simulink library "thermochemical"  (R2017b)
settings: Solver=VariableStepAuto  StartTime=0.0  StopTime=10.0  RelTol=1e-3
values from neighbouring files (symbols this model uses):
  c = conversion_factors()    [blk_clausius_clapeyron.m]    (also in blk_clausius_clapeyron_no_popup.m; blk_cold_room_closed_dry_air.m; blk_reactor_BaCl2_NH3_no_walls.m; blk_reactor_BaCl2_NH3_no_walls_state_space.m)
  cp = metal.cp    [blk_wall_simple.m]    (also in get_metal_properties.m = 390)
  fluid = get_param(blk,'fluid')    [blk_thermodynamic_properties_nonsaturated.m]    (also in blk_thermodynamic_properties_nonsaturated_interpreted.m; blk_thermodynamic_properties_saturated.m; blk_thermodynamic_properties_saturated_interpreted.m; blk_thermodynamic_properties_saturated_mix.m)
  gas = get_material_properties(x.gasName)    [blk_reactor_BaCl2_NH3_cylindrical_no_walls_fun1.m]
  h = get_param(gcb,'ObjectParameters')    [get_param_eval.m]
  rho = metal.rho    [blk_wall_simple.m]    (also in get_metal_properties.m = 8940)
  s = solve(eq,dx,'ReturnConditions',true)    [LMTD_inv.m]    (also in blk_wall_simple.m = get_param_eval(blk,'s'))
  u_gas_at_T_ref = -R * T_ref    [blk_reactor_BaCl2_NH3_no_walls.m]    (also in blk_reactor_BaCl2_NH3_no_walls_state_space.m)
undefined symbols (not defined in the file or in its folder): b_motor, BaCl2, beta, CoolProp, cP_binder, cP_gas, cP_s0, cv, dh_r_0, ENG, heat_exchanger_epsilonNTU_inv_simulink, heat_exchanger_epsilonNTU_simulink, J_motor, K_cin, kappa, Km_motor, La_motor, lookup2D_BreakPoint2, M_binder, N_binder, N_gas_free_volume_init, N_salt, NH3, nh3_v3, nu, P, phase, PID_D_motor, PID_I_motor, PID_P_motor, Ra_motor, Reactor_phase, T, T1, T2, T_init, Tr_init, Tr_ref, U_binder_at_Tr_ref, U_salt_at_X0_Tr_ref, Ur_init, V_void, Valve_regime, Vmax_motor, w_init_motor, X_init
libraries: thermochemical x247, simulink x54, dspsigops x3
(part 6 of 12)

== system thermochemical/Walls/Radial thermal resistance (no energy accumulation) ==
  In3 : Inport
  In1 : Inport  Port=2
  In2 : Inport  Port=3
  In4 : Inport  Port=4
  Divide : Product  Inputs=*/
  Divide1 : Product  Inputs=*/
  Gain2 : Gain  Gain=2*pi
  Math Function : Math  Operator=log  SaturateOnIntegerOverflow=on
  Product : Product  Inputs=**
  Out3 : Outport
  wires:
  Math Function/1 -> Divide/1
  Divide1/1 -> Math Function/1
  In1/1 -> Divide1/2  "Dinner (m)"
  In3/1 -> Product/1  "lambda (W/K/m)"
  Divide/1 -> Out3/1  "R (K/W)"
  In2/1 -> Divide1/1  "Douter (m)"
  In4/1 -> Product/2  "L (m)"
  Product/1 -> Gain2/1
  Gain2/1 -> Divide/2

== system thermochemical/Walls/Wall, simple, h as inputs ==
  note: Convective heat transfer.
      | Wall - Inner interface
  note: Wall, internal energy's
      | differential equation
  note: Convective heat transfer.
      | Wall - Outer interface
  In1 : Inport
  In3 : Inport  Port=2
  In2 : Inport  Port=3
  In4 : Inport  Port=4
  Gain1 : Gain  Gain=s
  Gain12 : Gain  Gain=s
  Gain14 : Gain  Gain=1/(e_mm*1e-3*s*rho*cp)
  Initial condition : Constant  Value=Twall_init
  Integrator4 : Integrator  InitialConditionSource=external  InitialCondition=T_init
  Product : Product
  Product1 : Product
  Sum13 : Sum  Inputs=|-+
  Sum15 : Sum  Inputs=-+
  Sum18 : Sum  Inputs=-+|
  Out2 : Outport
  Out1 : Outport  Port=2
  Out3 : Outport  Port=3
  wires:
  Product/1 -> Gain12/1
  In3/1 -> Product/1  "h outer (W/m²/K)"
  Initial condition/1 -> Integrator4/2
  Sum15/1 -> Gain14/1
  In1/1 -> Sum13/1  "T outer (K)"
  Gain12/1 -> Out3/1, Sum15/1  "Q wall → outer (W)"
  Integrator4/1 -> Sum18/1, Sum13/2, Out2/1  "T wall (K)"
  Sum18/1 -> Product1/1
  Gain1/1 -> Sum15/2, Out1/1  "Q inner → wall (W)"
  Sum13/1 -> Product/2
  Gain14/1 -> Integrator4/1  "dT/dt"
  In2/1 -> Sum18/2  "T inner (K)"
  Product1/1 -> Gain1/1
  In4/1 -> Product1/2  "h inner (W/m²/K)"

== system thermochemical/Walls/Wall, tube with//without fins ==
  note: Convective heat transfer.
      | Wall - Outer interface
  note: Internal energy's
      | differential equation
  note: Convective heat transfer.
      | Wall - Inner interface
  In1 : Inport
  In4 : Inport  Port=2
  In2 : Inport  Port=3
  In5 : Inport  Port=4
  Divide : Product  Inputs=*/
  Initial condition : Constant  Value=Tinit
  Integrator4 : Integrator  InitialConditionSource=external  InitialCondition=T_init
  Product : Product  Inputs=3
  Product1 : Product  Inputs=3
  Subsystem : Subsystem
  Subsystem1 : Subsystem
  Subsystem3 : Subsystem
  Sum13 : Sum  Inputs=|-+
  Sum15 : Sum  Inputs=-+
  Sum18 : Sum  Inputs=-+|
  s12 : Constant  Value=L_m
  s13 : Constant  Value=OD_mm
  s14 : Constant  Value=e_mm
  Out2 : Outport
  Out1 : Outport  Port=2
  Out3 : Outport  Port=3
  Out4 : Outport  Port=4
  wires:
  In2/1 -> Sum18/2  "T inner (K)"
  Divide/1 -> Integrator4/1  "dT/dt"
  Sum13/1 -> Product/3
  Product1/1 -> Sum15/2, Out1/1  "Q inner → wall (W)"
  Sum18/1 -> Product1/1
  Integrator4/1 -> Out2/1, Sum13/2, Sum18/1  "T wall (K)"
  Product/1 -> Sum15/1, Out3/1  "Q wall → outer (W)"
  In1/1 -> Sum13/1  "T outer (K)"
  Sum15/1 -> Divide/1  "Q net"
  Initial condition/1 -> Integrator4/2
  Subsystem3/2(Total tube effective finned area (m2)) -> Product/1
  In5/1 -> Product1/2  "h inner (W/m²/K)"
  In4/1 -> Subsystem3/1(In4), Product/2  "h outer (W/m²/K)"
  s13/1 -> Subsystem/1(In1)
  s14/1 -> Subsystem/2(In2)
  s12/1 -> Subsystem/3(In3)
  Subsystem/1(Inner area (m2)) -> Product1/3
  Subsystem1/1((m*Cp) fins + (m*Cp) tube) -> Divide/2
  Subsystem3/1(Total tube effective finned area (m2)1) -> Out4/1  "eta_fin (0..1)"

== system thermochemical/Walls/Wall, tube with//without fins, with internal heat production ==
  note: Convective heat transfer.
      | Wall - Inner interface
  note: Internal energy's
      | differential equation
  note: Convective heat transfer.
      | Wall - Outer interface
  In1 : Inport
  In4 : Inport  Port=2
  In2 : Inport  Port=3
  In5 : Inport  Port=4
  In3 : Inport  Port=5
  Divide : Product  Inputs=*/
  Initial condition : Constant  Value=Tinit
  Integrator4 : Integrator  InitialConditionSource=external  InitialCondition=T_init
  Product : Product  Inputs=3
  Product1 : Product  Inputs=3
  Subsystem : Subsystem
  Subsystem1 : Subsystem
  Subsystem3 : Subsystem
  Sum13 : Sum  Inputs=|-+
  Sum15 : Sum  Inputs=-++
  Sum18 : Sum  Inputs=-+|
  s12 : Constant  Value=L_m
  s13 : Constant  Value=OD_mm
  s14 : Constant  Value=e_mm
  Out2 : Outport
  Out1 : Outport  Port=2
  Out3 : Outport  Port=3
  Out4 : Outport  Port=4
  wires:
  Subsystem3/1(Total tube effective finned area (m2)1) -> Out4/1  "eta_fin (0..1)"
  Subsystem1/1((m*Cp) fins + (m*Cp) tube) -> Divide/2
  Subsystem/1(Inner area (m2)) -> Product1/3
  s12/1 -> Subsystem/3(In3)
  s14/1 -> Subsystem/2(In2)
  s13/1 -> Subsystem/1(In1)
  In4/1 -> Product/2, Subsystem3/1(In4)  "h outer (W/m²/K)"
  In5/1 -> Product1/2  "h inner (W/m²/K)"
  Subsystem3/2(Total tube effective finned area (m2)) -> Product/1
  Initial condition/1 -> Integrator4/2
  Sum15/1 -> Divide/1  "Q net"
  In1/1 -> Sum13/1  "T outer (K)"
  Product/1 -> Sum15/1, Out3/1  "Q wall → outer (W)"
  Integrator4/1 -> Sum18/1, Sum13/2, Out2/1  "T wall (K)"
  Sum18/1 -> Product1/1
  Product1/1 -> Sum15/3, Out1/1  "Q inner → wall (W)"
  Sum13/1 -> Product/3
  Divide/1 -> Integrator4/1  "dT/dt"
  In2/1 -> Sum18/2  "T inner (K)"
  In3/1 -> Sum15/2  "Q production (W)"

== system thermochemical/Compression/Gas compressor without motor/Compressor's power dW ==
  In1 : Inport
  In7 : Inport  Port=2
  In2 : Inport  Port=3
  Divide1 : Product  Inputs=**
  Sum2 : Sum  Inputs=-+
  Out2 : Outport
  wires:
  Sum2/1 -> Divide1/1  "delta h"
  In1/1 -> Sum2/2  "h_out (J/mol)"
  In7/1 -> Sum2/1  "h_in (J/mol)"
  In2/1 -> Divide1/2  "dn (mol/sec)"
  Divide1/1 -> Out2/1  "dW/dt compr. (W)"

== system thermochemical/Compression/Gas compressor without motor/Cp//Cv ==
  In1 : Inport
  In2 : Inport  Port=2
  Divide : Product  Inputs=*/
  Thermodynamic property (non-saturated) : thermochemical/Thermodynamic fluid properties/Thermodynamic  property (non-saturated)  sel=cp(T,P)  fluid=fluid  reciprocVar=-1  lookup2D_BreakPoint1=fluid.no_sat.T_P_indep.var_indep.T  lookup2D_BreakPoint2=fluid.no_sat.T_P_indep.var_indep.P  lookup2D_Data=fluid.no_sat.T_P_indep.var_dep.Cp_molar
      settings: SourceProductName=@ Thermochemical
  Thermodynamic property (non-saturated)1 : thermochemical/Thermodynamic fluid properties/Thermodynamic  property (non-saturated)  sel=cv(T,P)  fluid=fluid  reciprocVar=-1  lookup2D_BreakPoint1=fluid.no_sat.T_P_indep.var_indep.T  lookup2D_BreakPoint2=fluid.no_sat.T_P_indep.var_indep.P  lookup2D_Data=fluid.no_sat.T_P_indep.var_dep.Cv_molar
      settings: SourceProductName=@ Thermochemical
  Out1 : Outport
  wires:
  Thermodynamic property (non-saturated)/1 -> Divide/1
  Divide/1 -> Out1/1  "gamma (1)"
  In1/1 -> Thermodynamic property (non-saturated)1/1, Thermodynamic property (non-saturated)/1  "T (K)"
  Thermodynamic property (non-saturated)1/1 -> Divide/2
  In2/1 -> Thermodynamic property (non-saturated)1/2, Thermodynamic property (non-saturated)/2  "P (bar)"

== system thermochemical/Compression/Gas compressor without motor/Gas flow rate ==
  In2 : Inport
  In7 : Inport  Port=2
  In1 : Inport  Port=3
  In6 : Inport  Port=4
  Divide2 : Product  Inputs=**
  Divide3 : Product  Inputs=**
  Gain : Gain  Gain=3600
  Swept volume per radian (m3/rad) : Gain  Gain=dVswept_m3_h / dVswept_rmp / (2*pi*60)
  Terminator : Terminator
  Thermodynamic property (non-saturated) : thermochemical/Thermodynamic fluid properties/Thermodynamic  property (non-saturated)  sel=rho(T,P)  fluid=fluid  reciprocVar=-1  lookup2D_BreakPoint1=fluid.no_sat.T_P_indep.var_indep.T  lookup2D_BreakPoint2=fluid.no_sat.T_P_indep.var_indep.P  lookup2D_Data=fluid.no_sat.T_P_indep.var_dep.rho_molar
      settings: SourceProductName=@ Thermochemical
  Thermodynamic property (non-saturated)1 : thermochemical/Thermodynamic fluid properties/Thermodynamic  property (non-saturated)  sel=phase(T,P)  fluid=fluid  reciprocVar=-1  lookup2D_BreakPoint1=fluid.no_sat.T_P_indep.var_indep.T  lookup2D_BreakPoint2=fluid.no_sat.T_P_indep.var_indep.P  lookup2D_Data=fluid.no_sat.T_P_indep.var_dep.phase
      settings: SourceProductName=@ Thermochemical
  Out2 : Outport
  Out1 : Outport  Port=2
  Out3 : Outport  Port=3
  Out4 : Outport  Port=4
  wires:
  Divide2/1 -> Out2/1  "dn/dt (mol/sec)"
  In6/1 -> Divide3/2  "eta vol ([0..1])"
  Divide3/1 -> Divide2/1, Out1/1  "dV/dt effective (m3/sec)"
  In1/1 -> Swept volume per radian (m3/rad)/1  "omega (rad/sec)"
  Swept volume per radian (m3/rad)/1 -> Gain/1, Divide3/1, Out3/1  "dV/dt swept (m3/sec)"
  In7/1 -> Thermodynamic property (non-saturated)1/2, Thermodynamic property (non-saturated)/2  "P in (bar)"
  Thermodynamic property (non-saturated)/1 -> Divide2/2  "rho_gas (mol/m3)"
  In2/1 -> Thermodynamic property (non-saturated)1/1, Thermodynamic property (non-saturated)/1  "T in (K)"
  Gain/1 -> Out4/1  "dV/dt swept (m3/h)"
  Thermodynamic property (non-saturated)1/1 -> Terminator/1  "phase"

== system thermochemical/Compression/Gas compressor without motor/Torque  ==
  In5 : Inport
  In8 : Inport  Port=2
  In6 : Inport  Port=3
  In2 : Inport  Port=4
  In7 : Inport  Port=5
  Divide2 : Product  Inputs=****
  Gain5 : Gain  Gain=1/eta_mech
  Sum2 : Sum  Inputs=-+
  Swept volume per radian (m3/rad) : Constant  Value=dVswept_m3_h / dVswept_rmp / (2*pi*60)
  Thermodynamic property (non-saturated) : thermochemical/Thermodynamic fluid properties/Thermodynamic  property (non-saturated)  sel=rho(T,P)  fluid=fluid  reciprocVar=-1  lookup2D_BreakPoint1=fluid.no_sat.T_P_indep.var_indep.T  lookup2D_BreakPoint2=fluid.no_sat.T_P_indep.var_indep.P  lookup2D_Data=fluid.no_sat.T_P_indep.var_dep.rho_molar
      settings: SourceProductName=@ Thermochemical
  Out4 : Outport
  wires:
  In6/1 -> Divide2/3  "eta_vol ([0..1])"
  Thermodynamic property (non-saturated)/1 -> Divide2/4  "rho_gas (mol/m3)"
  Gain5/1 -> Out4/1  "Torque (Nm or J/rad)"
  Sum2/1 -> Divide2/2  "delta h (J/mol)"
  In5/1 -> Sum2/2  "h_out (J/mol)"
  In8/1 -> Sum2/1  "h_in (J/mol)"
  Divide2/1 -> Gain5/1
  In7/1 -> Thermodynamic property (non-saturated)/2  "P_in (bar)"
  In2/1 -> Thermodynamic property (non-saturated)/1  "T_in (K)"
  Swept volume per radian (m3/rad)/1 -> Divide2/1

== system thermochemical/Compression/Gas compressor without motor/Torque saturation towards zero speed (unidirectinal saturation) ==
  In2 : Inport
  In1 : Inport  Port=2
  Constant : Constant  Value=threshold  VectorParams1D=off
  Divide : Product  Inputs=/*
  Mult. : Product  Inputs=**
  Mux2 : Mux  Inputs=2
  Saturation : Saturate  UpperLimit=1  LowerLimit=output_min
  Saturation1 : Saturate  UpperLimit=Inf  LowerLimit=0
  Terminator : Terminator
  Out1 : Outport
  wires:
  In2/1 -> Saturation1/1  "input"
  Divide/1 -> Saturation/1
  Saturation/1 -> Mult./2
  Constant/1 -> Divide/1
  Mult./1 -> Mux2/2, Out1/1  "output"
  Mux2/1 -> Terminator/1
  In1/1 -> Divide/2  "control"
  Saturation1/1 -> Mux2/1, Mult./1

== system thermochemical/Compression/Gas compressor without motor/Volumetric efficiency (pesimistic) ==
  In3 : Inport
  In4 : Inport  Port=2
  Constant : Constant
  Divide1 : Product  Inputs=*/
  Gain2 : Gain  Gain=CL
  Sum1 : Sum  Inputs=|-+
  Out5 : Outport
  wires:
  In4/1 -> Divide1/1  "HP (bar)"
  In3/1 -> Divide1/2  "LP (bar)"
  Divide1/1 -> Gain2/1  "compression_ratio"
  Constant/1 -> Sum1/2
  Gain2/1 -> Sum1/1
  Sum1/1 -> Out5/1  "nu_Vol"

== system thermochemical/Compression/Gas compressor without motor, two stages, ideal compression ratios/Compressor power ==
  In8 : Inport
  In5 : Inport  Port=2
  In3 : Inport  Port=3
  In1 : Inport  Port=4
  In2 : Inport  Port=5
  Divide1 : Product  Inputs=**
  Sum1 : Sum  Inputs=-+
  Sum2 : Sum  Inputs=-+
  Sum3 : Sum
  Out4 : Outport
  wires:
  Divide1/1 -> Out4/1  "dW/dt compr. (W)"
  Sum3/1 -> Divide1/1  "delta h (1st + 2nd stage) (J/mol)"
  In5/1 -> Sum2/2  "h out 1st stage (J/mol)"
  In8/1 -> Sum2/1  "h in 1st stage (J/mol)"
  In2/1 -> Divide1/2  "dn (mol/sec)"
  In3/1 -> Sum1/1  "h in 2nd stage (J/mol)"
  In1/1 -> Sum1/2  "h out 2nd stage (J/mol)"
  Sum1/1 -> Sum3/2
  Sum2/1 -> Sum3/1

== system thermochemical/Compression/Gas compressor without motor, two stages, ideal compression ratios/Cp//Cv ==
  In1 : Inport
  In2 : Inport  Port=2
  Divide : Product  Inputs=*/
  Thermodynamic property (non-saturated) : thermochemical/Thermodynamic fluid properties/Thermodynamic  property (non-saturated)  sel=cp(T,P)  fluid=fluid  reciprocVar=-1  lookup2D_BreakPoint1=fluid.no_sat.T_P_indep.var_indep.T  lookup2D_BreakPoint2=fluid.no_sat.T_P_indep.var_indep.P  lookup2D_Data=fluid.no_sat.T_P_indep.var_dep.Cp_molar
      settings: SourceProductName=@ Thermochemical
  Thermodynamic property (non-saturated)1 : thermochemical/Thermodynamic fluid properties/Thermodynamic  property (non-saturated)  sel=cv(T,P)  fluid=fluid  reciprocVar=-1  lookup2D_BreakPoint1=fluid.no_sat.T_P_indep.var_indep.T  lookup2D_BreakPoint2=fluid.no_sat.T_P_indep.var_indep.P  lookup2D_Data=fluid.no_sat.T_P_indep.var_dep.Cv_molar
      settings: SourceProductName=@ Thermochemical
  Out1 : Outport
  wires:
  Thermodynamic property (non-saturated)/1 -> Divide/1
  Divide/1 -> Out1/1  "gamma"
  In1/1 -> Thermodynamic property (non-saturated)1/1, Thermodynamic property (non-saturated)/1  "T (K)"
  Thermodynamic property (non-saturated)1/1 -> Divide/2
  In2/1 -> Thermodynamic property (non-saturated)1/2, Thermodynamic property (non-saturated)/2  "P (bar)"

== system thermochemical/Compression/Gas compressor without motor, two stages, ideal compression ratios/Gas flow rate ==
  In2 : Inport
  In7 : Inport  Port=2
  In1 : Inport  Port=3
  In6 : Inport  Port=4
  Divide2 : Product  Inputs=**
  Divide3 : Product  Inputs=**
  Gain : Gain  Gain=3600
  Swept volume per radian (m3/rad) : Gain  Gain=dVswept_m3_h / dVswept_rmp / (2*pi*60)
  Terminator : Terminator
  Thermodynamic property (non-saturated) : thermochemical/Thermodynamic fluid properties/Thermodynamic  property (non-saturated)  sel=rho(T,P)  fluid=fluid  reciprocVar=-1  lookup2D_BreakPoint1=fluid.no_sat.T_P_indep.var_indep.T  lookup2D_BreakPoint2=fluid.no_sat.T_P_indep.var_indep.P  lookup2D_Data=fluid.no_sat.T_P_indep.var_dep.rho_molar
      settings: SourceProductName=@ Thermochemical
  Thermodynamic property (non-saturated)1 : thermochemical/Thermodynamic fluid properties/Thermodynamic  property (non-saturated)  sel=phase(T,P)  fluid=fluid  reciprocVar=-1  lookup2D_BreakPoint1=fluid.no_sat.T_P_indep.var_indep.T  lookup2D_BreakPoint2=fluid.no_sat.T_P_indep.var_indep.P  lookup2D_Data=fluid.no_sat.T_P_indep.var_dep.phase
      settings: SourceProductName=@ Thermochemical
  Out2 : Outport
  Out1 : Outport  Port=2
  Out3 : Outport  Port=3
  Out4 : Outport  Port=4
  wires:
  Divide2/1 -> Out2/1  "dn/dt (mol/sec)"
  In6/1 -> Divide3/2  "eta vol ([0..1])"
  Divide3/1 -> Divide2/1, Out1/1  "dV/dt effective (m3/sec)"
  In1/1 -> Swept volume per radian (m3/rad)/1  "omega (rad/sec)"
  Swept volume per radian (m3/rad)/1 -> Gain/1, Divide3/1, Out3/1  "dV/dt swept (m3/sec)"
  In7/1 -> Thermodynamic property (non-saturated)1/2, Thermodynamic property (non-saturated)/2  "P in (bar)"
  Thermodynamic property (non-saturated)/1 -> Divide2/2  "rho_gas (mol/m3)"
  In2/1 -> Thermodynamic property (non-saturated)1/1, Thermodynamic property (non-saturated)/1  "T in (K)"
  Gain/1 -> Out4/1  "dV/dt swept (m3/h)"
  Thermodynamic property (non-saturated)1/1 -> Terminator/1  "phase"

== system thermochemical/Compression/Gas compressor without motor, two stages, ideal compression ratios/Inter-stage pressure ==
  In1 : Inport
  In7 : Inport  Port=2
  In2 : Inport  Port=3
  Constant : Constant  Value=0.5
  Divide1 : Product  Inputs=*/
  Divide2 : Product  Inputs=*/
  Divide3 : Product  Inputs=*/
  Math Function : Math  Operator=pow  SaturateOnIntegerOverflow=on
  Out2 : Outport
  wires:
  Math Function/1 -> Divide3/2  "CR1"
  Divide2/1 -> Math Function/1  "CR1²"
  Divide1/1 -> Divide2/1  "CR"
  Constant/1 -> Math Function/2
  Divide3/1 -> Out2/1  "P interm. (bar)"
  In2/1 -> Divide2/2  "CR2 / CR1"
  In7/1 -> Divide1/2  "P low (bar)"
  In1/1 -> Divide1/1, Divide3/1  "P high (bar)"

== system thermochemical/Compression/Gas compressor without motor, two stages, ideal compression ratios/Torque 1st stage 1 ==
  In8 : Inport
  In5 : Inport  Port=2
  In3 : Inport  Port=3
  In1 : Inport  Port=4
  In6 : Inport  Port=5
  In2 : Inport  Port=6
  In7 : Inport  Port=7
  Divide2 : Product  Inputs=****
  Gain5 : Gain  Gain=1/eta_mech
  Sum1 : Sum  Inputs=-+
  Sum2 : Sum  Inputs=-+
  Sum3 : Sum
  Swept volume per radian (m3/rad) : Constant  Value=dVswept_m3_h / dVswept_rmp / (2*pi*60)
  Thermodynamic property (non-saturated) : thermochemical/Thermodynamic fluid properties/Thermodynamic  property (non-saturated)  sel=rho(T,P)  fluid=fluid  reciprocVar=-1  lookup2D_BreakPoint1=fluid.no_sat.T_P_indep.var_indep.T  lookup2D_BreakPoint2=fluid.no_sat.T_P_indep.var_indep.P  lookup2D_Data=fluid.no_sat.T_P_indep.var_dep.rho_molar
      settings: SourceProductName=@ Thermochemical
  Out4 : Outport
  wires:
  Sum2/1 -> Sum3/1
  Sum1/1 -> Sum3/2
  In1/1 -> Sum1/2  "h out 2nd stage (J/mol)"
  In3/1 -> Sum1/1  "h in 2nd stage (J/mol)"
  Swept volume per radian (m3/rad)/1 -> Divide2/1
  In2/1 -> Thermodynamic property (non-saturated)/1  "T in 1st stage (K)"
  In7/1 -> Thermodynamic property (non-saturated)/2  "P in 1st stage (bar)"
  Divide2/1 -> Gain5/1
  In8/1 -> Sum2/1  "h in 1st stage (J/mol)"
  In5/1 -> Sum2/2  "h out 1st stage (J/mol)"
  Sum3/1 -> Divide2/2  "delta h (1st + 2nd stage) (J/mol)"
  Gain5/1 -> Out4/1  "Torque (Nm or J/rad)"
  Thermodynamic property (non-saturated)/1 -> Divide2/4  "rho_gas (mol/m3)"
  In6/1 -> Divide2/3  "eta_vol ([0..1])"

== system thermochemical/Compression/Gas compressor without motor, two stages, ideal compression ratios/Torque saturation towards zero speed (unidirectinal saturation) ==
  In2 : Inport
  In1 : Inport  Port=2
  Constant : Constant  Value=threshold  VectorParams1D=off
  Divide : Product  Inputs=/*
  Mult. : Product  Inputs=**
  Mux2 : Mux  Inputs=2
  Saturation : Saturate  UpperLimit=1  LowerLimit=output_min
  Saturation1 : Saturate  UpperLimit=Inf  LowerLimit=0
  Terminator : Terminator
  Out1 : Outport
  wires:
  In2/1 -> Saturation1/1  "input"
  Divide/1 -> Saturation/1
  Saturation/1 -> Mult./2
  Constant/1 -> Divide/1
  Mult./1 -> Mux2/2, Out1/1  "output"
  Mux2/1 -> Terminator/1
  In1/1 -> Divide/2  "control"
  Saturation1/1 -> Mux2/1, Mult./1

== system thermochemical/Compression/Gas compressor without motor, two stages, ideal compression ratios/Volumetric efficiency (pesimistic) ==
  In3 : Inport
  In4 : Inport  Port=2
  Constant : Constant
  Divide1 : Product  Inputs=*/
  Gain2 : Gain  Gain=CL
  Sum1 : Sum  Inputs=|-+
  Out5 : Outport
  wires:
  In4/1 -> Divide1/1  "HP (bar)"
  In3/1 -> Divide1/2  "LP (bar)"
  Divide1/1 -> Gain2/1  "compression_ratio"
  Constant/1 -> Sum1/2
  Gain2/1 -> Sum1/1
  Sum1/1 -> Out5/1  "nu_Vol"

== system thermochemical/Control volumes/Two-phase saturated fluid control volume (with wall, simple)/Subsystem2 ==
  In2 : Inport
  In3 : Inport  Port=2
  In1 : Inport  Port=3
  1 : Constant
  Product : Product
  Product1 : Product
  Sum11 : Sum  Inputs=+-|
  Sum9 : Sum  Inputs=|++
  Out1 : Outport
  wires:
  Sum9/1 -> Out1/1  "h equiv (W/m²/K)"
  In1/1 -> Product/2, Sum11/2  "liquid level (0..1)"
  In3/1 -> Product1/2  "h gas-wall (W/m²/K)"
  In2/1 -> Product/1  "h liquid-wall (W/m²/K)"
  Sum11/1 -> Product1/1  "gas level"
  1/1 -> Sum11/1
  Product1/1 -> Sum9/2  "h vap (W/m²/K)"
  Product/1 -> Sum9/1  "h liq (W/m²/K)"

== system thermochemical/Control volumes/Two-phase saturated fluid control volume (with wall, simple) (without algebraic loop)/Subsystem2 ==
  In2 : Inport
  In3 : Inport  Port=2
  In1 : Inport  Port=3
  1 : Constant
  Product : Product
  Product1 : Product
  Sum11 : Sum  Inputs=+-|
  Sum9 : Sum  Inputs=|++
  Out1 : Outport
  wires:
  Product/1 -> Sum9/1  "h liq (W/m²/K)"
  Product1/1 -> Sum9/2  "h vap (W/m²/K)"
  1/1 -> Sum11/1
  Sum11/1 -> Product1/1  "gas level"
  In2/1 -> Product/1  "h liquid-wall (W/m²/K)"
  In3/1 -> Product1/2  "h gas-wall (W/m²/K)"
  In1/1 -> Sum11/2, Product/2  "liquid level (0..1)"
  Sum9/1 -> Out1/1  "h equiv (W/m²/K)"

== system thermochemical/Control volumes/Two-phase saturated fluid control volume (with wall, tube with//without fins)/Subsystem2 ==
  In2 : Inport
  In3 : Inport  Port=2
  In1 : Inport  Port=3
  1 : Constant
  Mux : Mux  Inputs=2
  Product : Product
  Product1 : Product
  Scope1 : Scope
  Sum11 : Sum  Inputs=+-|
  Sum9 : Sum  Inputs=|++
  Out1 : Outport
  wires:
  Product/1 -> Mux/1, Sum9/1  "liquid"
  Product1/1 -> Mux/2, Sum9/2  "vapor"
  Mux/1 -> Scope1/1
  1/1 -> Sum11/1
  Sum11/1 -> Product1/1  "gas level"
  In2/1 -> Product/1  "h liquid-wall (W/m2/K)"
  In3/1 -> Product1/2  "h gas-wall (W/m2/K)"
  In1/1 -> Sum11/2, Product/2  "liquid level (0..1)"
  Sum9/1 -> Out1/1  "h equiv (W/m2/K)"

== system thermochemical/Control volumes/Two-phase saturated fluid control volume (with wall, tube with//without fins) (without algebraic loop)/Subsystem2 ==
  In2 : Inport
  In3 : Inport  Port=2
  In1 : Inport  Port=3
  1 : Constant
  Mux : Mux  Inputs=2
  Product : Product
  Product1 : Product
  Scope1 : Scope
  Sum11 : Sum  Inputs=+-|
  Sum9 : Sum  Inputs=|++
  Out1 : Outport
  wires:
  Sum9/1 -> Out1/1  "h equiv (W/m2/K)"
  In1/1 -> Product/2, Sum11/2  "liquid level (0..1)"
  In3/1 -> Product1/2  "h gas-wall (W/m2/K)"
  In2/1 -> Product/1  "h liquid-wall (W/m2/K)"
  Sum11/1 -> Product1/1  "gas level"
  1/1 -> Sum11/1
  Mux/1 -> Scope1/1
  Product1/1 -> Sum9/2, Mux/2  "vapor"
  Product/1 -> Sum9/1, Mux/1  "liquid"

== system thermochemical/Control volumes/Two-phase saturated fluid control volume (without walls)/Heat exchanger's temperature and liquid level ==
  In2 : Inport
  In1 : Inport  Port=2
  2 : Constant  Value=V
  Algebraic Constraint : AlgebraicConstraint  InitialGuess=T_init
  Check Dynamic Lower Bound : simulink/Model Verification/Check Dynamic  Lower Bound  Description=min < u  Enabled=on  stopWhenAssertionFail=on  export=off  icon=graphic
      settings: SourceProductName=Simulink  SourceProductBaseCode=SL
  Display : Display
  Scope9 : Scope
  Sum12 : Sum  Inputs=+-|
  Two-phase saturated fluid control volume energy equation : thermochemical/Control volumes/Two-phase saturated fluid control volume energy equation  fluid=fluid
      settings: SourceProductName=@ Thermochemical
  dn_gas1 : Constant  Value=fluid.constants.Tmin
  Out1 : Outport
  Out3 : Outport  Port=2
  Out2 : Outport  Port=3
  wires:
  Two-phase saturated fluid control volume energy equation/2 -> Out2/1  "liquid volumetric fraction (0..1)"
  Algebraic Constraint/1 -> Two-phase saturated fluid control volume energy equation/3, Check Dynamic Lower Bound/2, Out1/1  "T (K)"
  dn_gas1/1 -> Check Dynamic Lower Bound/1
  In2/1 -> Two-phase saturated fluid control volume energy equation/1  "N (mol)"
  In1/1 -> Sum12/1  "U (J)"
  Sum12/1 -> Scope9/1, Display/1, Algebraic Constraint/1  "error U"
  Two-phase saturated fluid control volume energy equation/1 -> Sum12/2
  Two-phase saturated fluid control volume energy equation/3 -> Out3/1  "vapor quality (0..1)"
  2/1 -> Two-phase saturated fluid control volume energy equation/2

== system thermochemical/Control volumes/Two-phase saturated fluid control volume (without walls)/Internal energy differential equation ==
  note: Internal energy's
      | differential equation
  In1 : Inport
  In2 : Inport  Port=2
  In3 : Inport  Port=3
  In5 : Inport  Port=4
  In4 : Inport  Port=5
  In7 : Inport  Port=6
  In6 : Inport  Port=7
  1 : Constant  Value=N_init
  2 : Constant  Value=T_init
  3 : Constant  Value=V
  HX energy rate balance : Subsystem
  Integrator2 : Integrator  InitialConditionSource=external
  Terminator : Terminator
  Terminator1 : Terminator
  Two-phase saturated fluid control volume energy equation : thermochemical/Control volumes/Two-phase saturated fluid control volume energy equation  fluid=fluid
      settings: SourceProductName=@ Thermochemical
  Out1 : Outport
  wires:
  Integrator2/1 -> Out1/1  "U hx (J)"
  In4/1 -> HX energy rate balance/5(In4)  "dn/dt vap,out (mol/sec)"
  In3/1 -> HX energy rate balance/3(In3)  "dn/dt in (mol/sec)"
  1/1 -> Two-phase saturated fluid control volume energy equation/1
  2/1 -> Two-phase saturated fluid control volume energy equation/3
  Two-phase saturated fluid control volume energy equation/1 -> Integrator2/2  "U hx init"
  3/1 -> Two-phase saturated fluid control volume energy equation/2
  Two-phase saturated fluid control volume energy equation/2 -> Terminator/1
  Two-phase saturated fluid control volume energy equation/3 -> Terminator1/1
  In6/1 -> HX energy rate balance/7(In6)  "dn/dt liq,out (mol/sec)"
  In1/1 -> HX energy rate balance/1(In1)  "q wall → hx (W)"
  In2/1 -> HX energy rate balance/2(In2)  "h in (J/mol)"
  In5/1 -> HX energy rate balance/4(In5)  "h vap (J/mol)"
  In7/1 -> HX energy rate balance/6(In7)  "h liq (J/mol)"
  HX energy rate balance/1(Out1) -> Integrator2/1

== system thermochemical/Control volumes/Two-phase saturated fluid control volume (without walls) (without algebraic loop)/Reactor output function ==
  In1 : Inport
  2 : Constant  Value=V
  Demux : Demux  Outputs=2
  Mux : Mux  Inputs=7
  Product : Product  Inputs=/*
  Thermodynamic property (saturated)1 : thermochemical/Thermodynamic fluid properties/Thermodynamic  property (saturated)  sel=h(T) vap. (J/mol)  fluid=fluid  lookup1D_BreakPoint1=fluid.sat.T  lookup1D_Data=fluid.sat.vap.h_molar
      settings: SourceProductName=@ Thermochemical
  Thermodynamic property (saturated)2 : thermochemical/Thermodynamic fluid properties/Thermodynamic  property (saturated)  sel=P(T) (bar)  fluid=fluid  lookup1D_BreakPoint1=fluid.sat.T  lookup1D_Data=fluid.sat.Psat
      settings: SourceProductName=@ Thermochemical
  Thermodynamic property (saturated)3 : thermochemical/Thermodynamic fluid properties/Thermodynamic  property (saturated)  sel=h(T) liq. (J/mol)  fluid=fluid  lookup1D_BreakPoint1=fluid.sat.T  lookup1D_Data=fluid.sat.liq.h_molar
      settings: SourceProductName=@ Thermochemical
  Thermodynamic property (saturated vapor-liquid mix) : thermochemical/Thermodynamic fluid properties/Thermodynamic property  (saturated vapor-liquid mix)  sel=h(T) (J/mol)  fluid=fluid  lookup1D_BreakPoint=0  lookup1D_Data1=fluid.sat.liq.h_molar  lookup1D_Data2=fluid.sat.vap.h_molar
      settings: SourceProductName=@ Thermochemical
  Vapor quality & Liquid volumetric fraction : thermochemical/Thermodynamic fluid properties/Vapor quality & Liquid  volumetric fraction  fluid=fluid
      settings: SourceProductName=@ Thermochemical
  Out1 : Outport
  wires:
  Demux/1 -> Thermodynamic property (saturated)3/1, Thermodynamic property (saturated vapor-liquid mix)/1, Thermodynamic property (saturated)1/1, Vapor quality & Liquid volumetric fraction/1, Mux/1, Thermodynamic property (saturated)2/1  "T (K)"
  Demux/2 -> Product/1  "v (m3/mol)"
  Mux/1 -> Out1/1  "Y(vector)"
  In1/1 -> Demux/1  "X(vector)"
  Vapor quality & Liquid volumetric fraction/1 -> Thermodynamic property (saturated vapor-liquid mix)/2, Mux/4  "vapor quality (0..1)"
  Thermodynamic property (saturated)1/1 -> Mux/5  "h vap (J/mol)"
  Vapor quality & Liquid volumetric fraction/2 -> Mux/3  "liquid volumetric fraction (0..1)"
  Thermodynamic property (saturated vapor-liquid mix)/1 -> Mux/6  "h liq+vap (J/mol)"
  Thermodynamic property (saturated)2/1 -> Mux/2  "P (bar)"
  Thermodynamic property (saturated)3/1 -> Mux/7  "h liq (J/mol)"
  Product/1 -> Vapor quality & Liquid volumetric fraction/2  "N (mol)"
  2/1 -> Vapor quality & Liquid volumetric fraction/3, Product/2

== system thermochemical/Control volumes/Two-phase saturated fluid control volume (without walls) (without algebraic loop)/Two-phase control volume state-space functions ==
  In1 : Inport
  In2 : Inport  Port=2
  Mux : Mux  Inputs=2
  f1 : Subsystem
  f2 : Subsystem
  Out2 : Outport
  wires:
  In2/1 -> f2/2(In2), f1/2(In1)  "U(vector)"
  In1/1 -> f2/1(In6), f1/1(In6)  "X(vector)"
  Mux/1 -> Out2/1  "dX/dt(vector)"
  f1/1(Out2) -> Mux/1
  f2/1(Out2) -> Mux/2

== system thermochemical/Conversions/Temperature conversion/Subsystem ==
  (K) : Inport
  Constant : Constant  Value=273.15
  Sum1 : Sum  Inputs=|+-
  (°C) : Outport
  wires:
  (K)/1 -> Sum1/1  "(K)"
  Sum1/1 -> (°C)/1  "(°C)"
  Constant/1 -> Sum1/2

== system thermochemical/Conversions/Temperature conversion/Subsystem1 ==
  (K) : Inport
  Constant : Constant  Value=273.15
  Sum1 : Sum  Inputs=|++
  (°C) : Outport
  wires:
  Constant/1 -> Sum1/2
  Sum1/1 -> (°C)/1  "(K)"
  (K)/1 -> Sum1/1  "(°C)"

== system thermochemical/Conversions/Temperature conversion/Subsystem2 ==
  (K) : Inport
  Constant : Constant  Value=32
  Gain : Gain  Gain=9/5
  Sum1 : Sum  Inputs=|++
  (°C) : Outport
  wires:
  (K)/1 -> Gain/1  "(°C)"
  Sum1/1 -> (°C)/1  "(°F)"
  Constant/1 -> Sum1/2
  Gain/1 -> Sum1/1

== system thermochemical/Conversions/Temperature conversion/Subsystem3 ==
  (K) : Inport
  Constant : Constant  Value=32
  Gain : Gain  Gain=5/9
  Sum1 : Sum  Inputs=|+-
  (°C) : Outport
  wires:
  Constant/1 -> Sum1/2
  Sum1/1 -> Gain/1
  (K)/1 -> Sum1/1  "(°F)"
  Gain/1 -> (°C)/1  "(°C)"

== system thermochemical/Conversions/Temperature conversion/Subsystem4 ==
  (K) : Inport
  Constant : Constant  Value=459.67
  Sum1 : Sum  Inputs=|++
  (°C) : Outport
  wires:
  Constant/1 -> Sum1/2
  Sum1/1 -> (°C)/1  "(°R)"
  (K)/1 -> Sum1/1  "(°F)"

== system thermochemical/Conversions/Temperature conversion/Subsystem5 ==
  (K) : Inport
  Constant : Constant  Value=459.67
  Sum1 : Sum  Inputs=|+-
  (°C) : Outport
  wires:
  (K)/1 -> Sum1/1  "(°R)"
  Sum1/1 -> (°C)/1  "(°F)"
  Constant/1 -> Sum1/2

== system thermochemical/Heat exchangers/Heat Exchanger, e-NTU method (UA input) Loop 2: water/Subsystem ==
  In1 : Inport
  In2 : Inport  Port=2
  In3 : Inport  Port=3
  In4 : Inport  Port=4
  In5 : Inport  Port=5
  In6 : Inport  Port=6
  In7 : Inport  Port=7
  NTU as a function of flow configuration : Subsystem
  Product1 : Product
  Product2 : Product
  Product3 : Product  Inputs=/*
  Subsystem1 : Subsystem
  Sum : Sum  Inputs=-+
  Q HX2 (W)9 : Outport
  Q HX2 (W)8 : Outport  Port=2
  Q HX2 (W)10 : Outport  Port=3
  Q HX2 (W)11 : Outport  Port=4
  Q HX2 (W)4 : Outport  Port=5
  Q HX2 (W)3 : Outport  Port=6
  Q HX2 (W)6 : Outport  Port=7
  wires:
  NTU as a function of flow configuration/1(Q HX2 (W)8) -> Product2/2, Q HX2 (W)8/1  "epsilon (0..1)"
  In5/1 -> Subsystem1/5(In5)  "dn/dt 2 (mol/sec)"
  In3/1 -> Subsystem1/3(In3)  "P1 in = P1 out (bar)"
  In4/1 -> Subsystem1/4(In4)  "dn/dt 1 (mol/sec)"
  In1/1 -> Subsystem1/1(In1), Sum/2  "T1 in (K)"
  In2/1 -> Subsystem1/2(In2)  "T1 out (K)"
  In7/1 -> Sum/1  "T2 in (K)"
  Subsystem1/4(Q HX2 (W)3) -> Q HX2 (W)6/1  "C2 (W/K)"
  Product1/1 -> Product2/1, Q HX2 (W)10/1  "q1→2 max (W)"
  Subsystem1/2(Q HX2 (W)7) -> Q HX2 (W)11/1, NTU as a function of flow configuration/1(In1)  "Cr (0..1)"
  Sum/1 -> Product1/1
  Subsystem1/1(Q HX2 (W)1) -> Product3/1, Product1/2  "Cmin (W/K)"
  Product2/1 -> Q HX2 (W)4/1  "q1→2 (W)"
  Subsystem1/3(Q HX2 (W)2) -> Q HX2 (W)3/1  "C1 (W/K)"
  In6/1 -> Product3/2  "UA (W/K)"
  Product3/1 -> Q HX2 (W)9/1, NTU as a function of flow configuration/2(In6)  "NTU (1)"

== system thermochemical/Heat exchangers/Heat Exchanger, e-NTU method (UA input) One fluid or condensation//evaporation Loop 2: water/NTU ==
  In6 : Inport
  Constant : Constant
  Gain : Gain  Gain=-1
  Math Function : Math  SaturateOnIntegerOverflow=on
  Sum : Sum  Inputs=+-|
  Q HX2 (W)8 : Outport
  wires:
  Constant/1 -> Sum/1
  In6/1 -> Gain/1  "NTU (1)"
  Sum/1 -> Q HX2 (W)8/1  "epsilon (0..1)"
  Math Function/1 -> Sum/2
  Gain/1 -> Math Function/1

== system thermochemical/Heat exchangers/Heat Exchanger, e-NTU method (epsilon input) Loop 2: water/Subsystem ==
  In1 : Inport
  In2 : Inport  Port=2
  In3 : Inport  Port=3
  In4 : Inport  Port=4
  In5 : Inport  Port=5
  In6 : Inport  Port=6
  In7 : Inport  Port=7
  NTU as a function of flow configuration : Subsystem
  Product : Product
  Product1 : Product
  Product2 : Product
  Subsystem1 : Subsystem
  Sum : Sum  Inputs=-+
  Q HX2 (W)8 : Outport
  Q HX2 (W)9 : Outport  Port=2
  Q HX2 (W)10 : Outport  Port=3
  Q HX2 (W)11 : Outport  Port=4
  Q HX2 (W)4 : Outport  Port=5
  Q HX2 (W)3 : Outport  Port=6
  Q HX2 (W)6 : Outport  Port=7
  wires:
  Subsystem1/3(Q HX2 (W)2) -> Q HX2 (W)3/1  "C1 (W/K)"
  Product2/1 -> Q HX2 (W)4/1  "q1→2 (W)"
  Subsystem1/1(Q HX2 (W)1) -> Product1/2, Product/1  "Cmin (W/K)"
  Sum/1 -> Product1/1
  Subsystem1/2(Q HX2 (W)7) -> NTU as a function of flow configuration/1(In1), Q HX2 (W)11/1  "Cr (0..1)"
  Product1/1 -> Q HX2 (W)10/1, Product2/2  "q1→2 max (W)"
  Product/1 -> Q HX2 (W)9/1  "UA (W/K)"
  Subsystem1/4(Q HX2 (W)3) -> Q HX2 (W)6/1  "C2 (W/K)"
  In7/1 -> Sum/1  "T2 in (K)"
  In2/1 -> Subsystem1/2(In2)  "T1 out (K)"
  In1/1 -> Sum/2, Subsystem1/1(In1)  "T1 in (K)"
  In4/1 -> Subsystem1/4(In4)  "dn/dt 1 (mol/sec)"
  In3/1 -> Subsystem1/3(In3)  "P1 in = P1 out (bar)"
  In5/1 -> Subsystem1/5(In5)  "dn/dt 2 (mol/sec)"
  In6/1 -> NTU as a function of flow configuration/2(In6), Product2/1  "epsilon (0..1)"
  NTU as a function of flow configuration/1(Q HX2 (W)8) -> Product/2, Q HX2 (W)8/1  "NTU (1)"

== system thermochemical/Heat exchangers/Heat Exchanger, e-NTU method (epsilon input) One fluid or condensation//evaporation Loop 2: water/NTU ==
  In6 : Inport
  Constant : Constant
  Gain : Gain  Gain=-1
  Math Function : Math  Operator=log  SaturateOnIntegerOverflow=on
  Sum : Sum  Inputs=+-|
  Q HX2 (W)8 : Outport
  wires:
  Gain/1 -> Q HX2 (W)8/1  "NTU (1)"
  In6/1 -> Sum/2  "epsilon (0..1)"
  Constant/1 -> Sum/1
  Sum/1 -> Math Function/1
  Math Function/1 -> Gain/1

== system thermochemical/Heat exchangers/LMTD/ERROR DETECTION ==
  In2 : Inport
  In1 : Inport  Port=2
  Constant : Constant
  Product : Product
  Sign : Signum
  Sign1 : Signum
  Sum : Sum  Inputs=|++
  Out2 : Outport
  wires:
  Sign/1 -> Product/1
  Product/1 -> Sum/1
  In1/1 -> Sign1/1  "signal 2"
  Constant/1 -> Sum/2
  Sum/1 -> Out2/1  "Result is zero  if signals have different sign"
  In2/1 -> Sign/1  "signal 1"
  Sign1/1 -> Product/2

== system thermochemical/Motors/DC motor + DC power supply + speed controller/DC Power source, limited in its maximum instantaneous power ==
  In3 : Inport
  In2 : Inport  Port=2
  In1 : Inport  Port=3
  Abs : Abs
  Constant : Constant
  Constant1 : Constant  Value=0
  Product : Product
  Product1 : Product  Inputs=*/
  Sum : Sum  Inputs=-+
  Switch : Switch  Criteria=u2 > Threshold
  Switch1 : Switch  Criteria=u2 > Threshold
  Out1 : Outport
  Out2 : Outport  Port=2
  wires:
  In2/1 -> Switch/3, Product/2  "U ref (V)"
  In1/1 -> Product1/2, Product/1  "I load (A)"
  Switch/1 -> Out1/1  "U power source (V)"
  In3/1 -> Product1/1, Sum/1  "Pow max (W)"
  Switch1/1 -> Out2/1  "Power clamp (0/1)"
  Product/1 -> Abs/1
  Abs/1 -> Sum/2
  Sum/1 -> Switch1/2, Switch/2
  Product1/1 -> Switch/1  "U clamp"
  Constant/1 -> Switch1/1  "clamp"
  Constant1/1 -> Switch1/3  "no clamp"

== system thermochemical/Reactors/Reactor's internal energy equation/Binder ==
  In2 : Inport
  1 : Constant  Value=U_binder_at_Tr_ref
  3 : Constant  Value=Tr_ref
  Gain6 : Gain  Gain=N_binder * M_binder * cP_binder
  Sum1 : Sum  Inputs=|++
  Sum5 : Sum  Inputs=|+-
  Out1 : Outport
  wires:
  Sum1/1 -> Out1/1  "U binder (J)"
  In2/1 -> Sum5/1  "Tr (K)"
  3/1 -> Sum5/2
  Sum5/1 -> Gain6/1
  1/1 -> Sum1/2
  Gain6/1 -> Sum1/1

== system thermochemical/Reactors/Reactor's internal energy equation/Gas ==
  In2 : Inport
  In3 : Inport  Port=2
  3 : Constant  Value=is_ideal_gas_in_void_volume
  Gain1 : Gain  Gain=1/V_void
  Internal energy of ideal gas : thermochemical/Thermodynamic fluid properties/Internal energy of ideal gas  T_ref=Tr_ref  Cv_gas=cP_gas - R  u_gas_at_T_ref=u_gas_at_Tr_ref
      settings: SourceProductName=@ Thermochemical
  Product3 : Product
  Switch : Switch  Criteria=u2 > Threshold  ZeroCross=off
  Thermodynamic property (non-saturated) : thermochemical/Thermodynamic fluid properties/Thermodynamic  property (non-saturated)  sel=u(T,rho)  fluid=fluid  reciprocVar=-1  lookup2D_BreakPoint1=fluid.no_sat.T_rho_indep.var_indep.T  lookup2D_BreakPoint2=fluid.no_sat.T_rho_indep.var_indep.rho_molar  lookup2D_Data=fluid.no_sat.T_rho_indep.var_dep.u_molar
      settings: SourceProductName=@ Thermochemical
  Out1 : Outport
  wires:
  In2/1 -> Internal energy of ideal gas/1, Thermodynamic property (non-saturated)/1  "Tr (K)"
  Thermodynamic property (non-saturated)/1 -> Switch/3  "u gas (real) (J/mol)"
  Internal energy of ideal gas/1 -> Switch/1  "u gas (ideal) (J/mol)"
  Product3/1 -> Out1/1  "U gas (J)"
  Gain1/1 -> Thermodynamic property (non-saturated)/2  "rho"
  Switch/1 -> Product3/1
  3/1 -> Switch/2
  In3/1 -> Product3/2, Gain1/1  "N_gas (void volume) (mol)"

== system thermochemical/Reactors/Reactor's internal energy equation/Salt ==
  In1 : Inport
  In2 : Inport  Port=2
  1 : Constant  Value=U_salt_at_X0_Tr_ref
  2 : Constant  Value=dh_r
  3 : Constant  Value=Tr_ref
  4 : Constant  Commented=on  Value=Tr_ref
  5 : Constant  Value=is_ideal_gas_in_salt
  Clausius-Clapeyron : thermochemical/Thermodynamic fluid properties/Clausius-Clapeyron  sel_1=P(T)  sel_2=BaCl2/NH3
      settings: SourceProductName=@ Thermochemical
  Clausius-Clapeyron1 : thermochemical/Thermodynamic fluid properties/Clausius-Clapeyron  Commented=on  sel_1=P(T)  sel_2=BaCl2/NH3
      settings: SourceProductName=@ Thermochemical
  Enthalpy of ideal gas : thermochemical/Thermodynamic fluid properties/Enthalpy of ideal gas  T_ref=Tr_ref  cP_gas=cP_gas  h_gas_at_T_ref=u_gas_at_Tr_ref + Tr_ref * R
      settings: SourceProductName=@ Thermochemical
  Gain1 : Gain  Gain=N_salt * nu
  Gain4 : Gain  Gain=N_salt * cP_s0
  Product2 : Product
  Sum1 : Sum  Inputs=+++
  Sum2 : Sum  Inputs=-+|
  Sum5 : Sum  Inputs=-+|
  Switch : Switch  Criteria=u2 > Threshold  ZeroCross=off
  Thermodynamic property (non-saturated) : thermochemical/Thermodynamic fluid properties/Thermodynamic  property (non-saturated)  sel=h(T,P)  fluid=fluid  reciprocVar=-1  lookup2D_BreakPoint1=fluid.no_sat.T_P_indep.var_indep.T  lookup2D_BreakPoint2=fluid.no_sat.T_P_indep.var_indep.P  lookup2D_Data=fluid.no_sat.T_P_indep.var_dep.h_molar
      settings: SourceProductName=@ Thermochemical
  Thermodynamic property (non-saturated)1 : thermochemical/Thermodynamic fluid properties/Thermodynamic  property (non-saturated)  Commented=on  sel=h(T,P)  fluid=fluid  reciprocVar=-1  lookup2D_BreakPoint1=fluid.no_sat.T_P_indep.var_indep.T  lookup2D_BreakPoint2=fluid.no_sat.T_P_indep.var_indep.P  lookup2D_Data=fluid.no_sat.T_P_indep.var_dep.h_molar
      settings: SourceProductName=@ Thermochemical
  Out1 : Outport
  wires:
  3/1 -> Sum5/1
  Sum1/1 -> Out1/1  "U salt (J)"
  In1/1 -> Gain1/1  "X [0..1]"
  Product2/1 -> Sum1/2
  Sum2/1 -> Product2/1
  Sum5/1 -> Gain4/1
  Gain1/1 -> Product2/2
  1/1 -> Sum1/3
  2/1 -> Sum2/1
  Gain4/1 -> Sum1/1
  Clausius-Clapeyron/1 -> Thermodynamic property (non-saturated)/2
  Clausius-Clapeyron1/1 -> Thermodynamic property (non-saturated)1/2
  4/1 -> Clausius-Clapeyron1/1, Thermodynamic property (non-saturated)1/1
  Thermodynamic property (non-saturated)/1 -> Switch/3  "h gas[Tr,Peq(Tr)] (J/mol)"
  Thermodynamic property (non-saturated)1/1 -> ?  "h gas[Tref,Peq(Tref)]"
  Switch/1 -> Sum2/2  "h gas(Tr)"
  Enthalpy of ideal gas/1 -> Switch/1  "h gas (ideal) (J/mol)"
  In2/1 -> Sum5/2, Clausius-Clapeyron/1, Thermodynamic property (non-saturated)/1, Enthalpy of ideal gas/1  "Tr (K)"
  5/1 -> Switch/2

== system thermochemical/Reactors/Reactor, BaCl2//NH3, state-space form, [Tr, Ng, X] as state variables, no algebraic loops, ideal gas in void volume, ideal gas in salt/Reactor, BaCl2, cylindrical, finned tube, state-space form, [Tr, Ng, X] as state variables, no algebraic loops, ideal gas in void volume ==
  In3 : Inport
  In1 : Inport  Port=2
  In2 : Inport  Port=3
  In4 : Inport  Port=4
  Display4 : Display
  Gain : Gain  Gain=-1
  "Reactor, BaCl2/NH3, cylindrical, no walls, state-space form, [Tr, Ng, X] as state variables, no algebraic loops, ideal gas in void volume" : thermochemical/Reactors/Reactor, BaCl2//NH3, state-space form, [Tr, Ng, X] as state variables, no algebraic loops, ideal gas in void volume, ideal gas in salt/Reactor, BaCl2//NH3, cylindrical, no walls, state-space form, [Tr, Ng, X] as state variables, no algebraic loops,  ideal gas in void volume  pairName=Barium chloride/Ammonia (BaCl2/NH3)  gasName=Ammonia gas (NH3)  binderName=ENG  tao_salt=0.75  rho_composite=300  K_cin=1e-3  fluid=nh3_v3  Lr=1.5  Lr_total=1.6  Dr=0.11  Ddiff=0.018  Tr_init=300  X_init=0.1  Vr_L=15.2053  m_composite_kg=4.162  m_salt_kg=3.1215  m_binder_kg=1.0405  m_gas_when_reactor_fully_charged_kg=2.0423  kWh_cold=0.77838  N_salt=14.9906  N_binder=86.6307  V_void=0.001332  N_gas_free_volume_init=0.16063
      settings: SourceProductName=@ Thermochemical
  "Wall, tube with/without fins" : thermochemical/Walls/Wall, tube with//without fins  L_m=1.6  OD_mm=114  e_mm=2  material_tube=Stainless steel AISI316  cp_tube=490.8  rho_tube=8023  height_fin_mm=0  thickness_fin_mm=0  pitch_fin_mm=0  material_fin=Steel  cp_fin=464.5  rho_fin=7847  lambda_fin=64.65  Tinit=300  mass_tube=4.5571  mass_fin=0  mass_total=4.5571  s_inner=0.56297  s_outer=0.57303
      settings: SourceProductName=@ Thermochemical
  composite-wall contact heat transfer coefficient (W/m2/K) : Constant  Value=300
  Out3 : Outport
  Out2 : Outport  Port=2
  Out4 : Outport  Port=3
  Out1 : Outport  Port=4
  Out5 : Outport  Port=5
  Out6 : Outport  Port=6
  Out7 : Outport  Port=7
  Out8 : Outport  Port=8
  wires:
  In4/1 -> "Reactor, BaCl2/NH3, cylindrical, no walls, state-space form, [Tr, Ng, X] as state variables, no algebraic loops, ideal gas in void volume"/2  "enthalpy in (J/mol) (only needed if dn/dt gas > 0)"
  In2/1 -> "Reactor, BaCl2/NH3, cylindrical, no walls, state-space form, [Tr, Ng, X] as state variables, no algebraic loops, ideal gas in void volume"/1  "dn/dt gas (mol/sec) > 0: gas in   < 0: gas out"
  "Wall, tube with/without fins"/1 -> Out3/1  "T wall (K)"
  "Reactor, BaCl2/NH3, cylindrical, no walls, state-space form, [Tr, Ng, X] as state variables, no algebraic loops, ideal gas in void volume"/2 -> Out4/1  "Pr (bar)"
  "Reactor, BaCl2/NH3, cylindrical, no walls, state-space form, [Tr, Ng, X] as state variables, no algebraic loops, ideal gas in void volume"/5 -> Out6/1  "X (0..1)"
  In1/1 -> "Wall, tube with/without fins"/2  "h outer (W/m2/K)"
  "Wall, tube with/without fins"/3 -> Out8/1  "Q wall → outer (W)"
  In3/1 -> "Wall, tube with/without fins"/1  "T outer (K)"
  "Reactor, BaCl2/NH3, cylindrical, no walls, state-space form, [Tr, Ng, X] as state variables, no algebraic loops, ideal gas in void volume"/3 -> Out1/1  "h gas (void space) (J/mol)"
  composite-wall contact heat transfer coefficient (W/m2/K)/1 -> "Wall, tube with/without fins"/4
  "Wall, tube with/without fins"/2 -> Out7/1, Gain/1  "Q inner → wall (W)"
  "Reactor, BaCl2/NH3, cylindrical, no walls, state-space form, [Tr, Ng, X] as state variables, no algebraic loops, ideal gas in void volume"/4 -> Out5/1  "Reaction phase"
  "Reactor, BaCl2/NH3, cylindrical, no walls, state-space form, [Tr, Ng, X] as state variables, no algebraic loops, ideal gas in void volume"/1 -> "Wall, tube with/without fins"/3, Out2/1  "Tr (K)"
  "Wall, tube with/without fins"/4 -> Display4/1
  Gain/1 -> "Reactor, BaCl2/NH3, cylindrical, no walls, state-space form, [Tr, Ng, X] as state variables, no algebraic loops, ideal gas in void volume"/3

== system thermochemical/Reactors/Reactor, BaCl2//NH3, state-space form, [Tr, Ng, X] as state variables, no algebraic loops, ideal gas in void volume, ideal gas in salt/Reactor, BaCl2//NH3, cylindrical, no walls, state-space form, [Tr, Ng, X] as state variables, no algebraic loops, ideal gas in void volume ==
  In3 : Inport
  In2 : Inport  Port=2
  In4 : Inport  Port=3
  "Reactor, BaCl2/NH3, no walls, state-space form, [Tr, Ng, X] as state variables, no algebraic loops, ideal gas in void volume" : thermochemical/Reactors/Reactor, BaCl2//NH3, state-space form, [Tr, Ng, X] as state variables, no algebraic loops, ideal gas in void volume, ideal gas in salt/Reactor, BaCl2//NH3, no walls, state-space form, [Tr, Ng, X] as state variables, no algebraic loops,  ideal gas in void volume  pairName=Barium chloride/Ammonia (BaCl2/NH3)  gasName=Ammonia gas (NH3)  binderName=ENG  N_salt=N_salt  N_binder=N_binder  K_cin=K_cin  V_void=V_void  fluid=fluid  Tr_init=Tr_init  X_init=X_init  N_gas_free_volume_init=N_gas_free_volume_init  m_composite_kg=4.1639  m_salt_kg=3.1235  m_binder_kg=1.0405  m_gas_when_reactor_fully_charged=2.0436  T_ref=300  u_gas_at_T_ref=0  U_binder_at_T_ref=0  U_salt_at_X0_T_ref=0  R=8.3145  cP_gas=42.5775  cV_gas=29.4370  nu=8  cP_s0=75.1  dh_r_0=38250  M_binder=0.012011  cP_binder=714.36  P_dead_zone=0.0001  dn_dead_zone=0.0001
      settings: SourceProductName=@ Thermochemical
  Out2 : Outport
  Out4 : Outport  Port=2
  Out3 : Outport  Port=3
  Out5 : Outport  Port=4
  Out1 : Outport  Port=5
  wires:
  In3/1 -> "Reactor, BaCl2/NH3, no walls, state-space form, [Tr, Ng, X] as state variables, no algebraic loops, ideal gas in void volume"/1  "dn/dt gas (mol/sec) > 0: gas in   < 0: gas out"
  In2/1 -> "Reactor, BaCl2/NH3, no walls, state-space form, [Tr, Ng, X] as state variables, no algebraic loops, ideal gas in void volume"/2  "enthalpy in (J/mol) (only needed if dn/dt gas > 0)"
  In4/1 -> "Reactor, BaCl2/NH3, no walls, state-space form, [Tr, Ng, X] as state variables, no algebraic loops, ideal gas in void volume"/3  "q out → in (W)"
  "Reactor, BaCl2/NH3, no walls, state-space form, [Tr, Ng, X] as state variables, no algebraic loops, ideal gas in void volume"/5 -> Out1/1  "X (0..1)"
  "Reactor, BaCl2/NH3, no walls, state-space form, [Tr, Ng, X] as state variables, no algebraic loops, ideal gas in void volume"/4 -> Out5/1  "Reaction phase"
  "Reactor, BaCl2/NH3, no walls, state-space form, [Tr, Ng, X] as state variables, no algebraic loops, ideal gas in void volume"/3 -> Out3/1  "h gas (void space) (J/mol)"
  "Reactor, BaCl2/NH3, no walls, state-space form, [Tr, Ng, X] as state variables, no algebraic loops, ideal gas in void volume"/2 -> Out4/1  "Pr (bar)"
  "Reactor, BaCl2/NH3, no walls, state-space form, [Tr, Ng, X] as state variables, no algebraic loops, ideal gas in void volume"/1 -> Out2/1  "Tr (K)"

== system thermochemical/Reactors/Reactor, BaCl2//NH3, state-space form, [Tr, Ng, X] as state variables, no algebraic loops, ideal gas in void volume, ideal gas in salt/Reactor, BaCl2//NH3, no walls, state-space form, [Tr, Ng, X] as state variables, no algebraic loops, ideal gas in void volume ==
  In3 : Inport
  In2 : Inport  Port=2
  In4 : Inport  Port=3
  "Reactor, no walls, state space form" : Subsystem
  Out2 : Outport
  Out1 : Outport  Port=2
  Out5 : Outport  Port=3
  Out3 : Outport  Port=4
  Out4 : Outport  Port=5
  wires:
  "Reactor, no walls, state space form"/1(X (0..1)) -> Out2/1  "Tr (K)"
  "Reactor, no walls, state space form"/3(P_reactor (bar)) -> Out4/1  "X (0..1)"
  "Reactor, no walls, state space form"/5(h_reactor_free_volume (J/mol)) -> Out3/1  "Reaction phase"
  "Reactor, no walls, state space form"/4(T_reactor (K)) -> Out5/1  "h gas void space (J/mol)"
  "Reactor, no walls, state space form"/2(Reactor phase) -> Out1/1  "Pr (bar)"
  In4/1 -> "Reactor, no walls, state space form"/1(q reactor → wall (W))  "q out → in (W)"
  In2/1 -> "Reactor, no walls, state space form"/3(In3)  "enthalpy in (J/mol) (only needed if dn/dt gas > 0)"
  In3/1 -> "Reactor, no walls, state space form"/2(enthalpy_in (J/mol) (only if dn_gas > 0))  "dn/dt gas (mol/sec) > 0: gas in   < 0: gas out"
